simulink model "SwingUp_LQR"  (R2016a)
settings: Solver=VariableStepAuto  StartTime=0.0  StopTime=30  RelTol=1e-3
undefined symbols (not defined in the file): K1, K2, K3, K4
libraries: simulink x2, instrumentlib x2
settings Model: Creator=VILLOTA  LastModifiedBy=VILLOTA

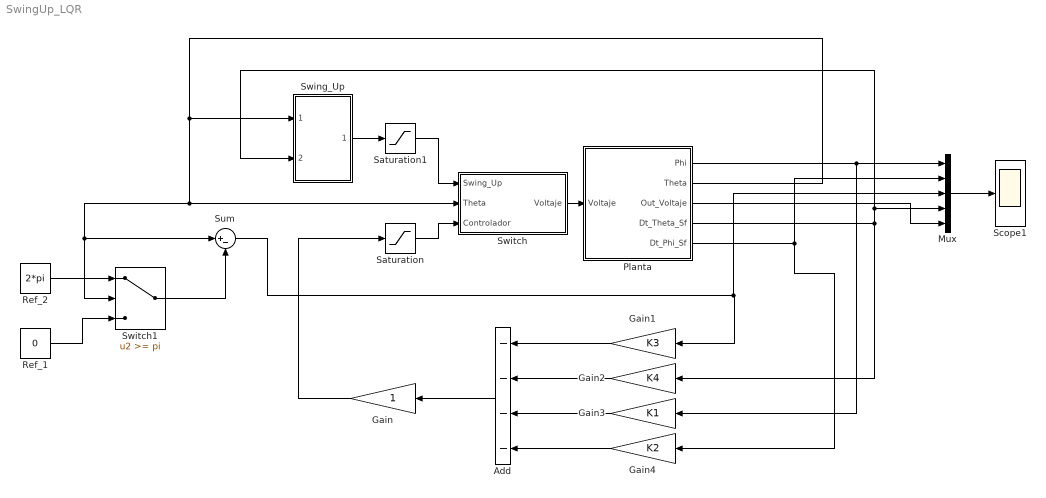
== system SwingUp_LQR ==
  Add : Sum  Inputs=----
  Gain : Gain
  Gain1 : Gain  Gain=K3
  Gain2 : Gain  Gain=K4
  Gain3 : Gain  Gain=K1
  Gain4 : Gain  Gain=K2
  Mux : Mux  Inputs=5
  Planta : Subsystem
  Ref_1 : Constant  Value=0
  Ref_2 : Constant  Value=2*pi
  Saturation : Saturate  UpperLimit=5  LowerLimit=-5
  Saturation1 : Saturate  UpperLimit=5  LowerLimit=-5
  Scope1 : Scope
  Sum : Sum  Inputs=|+-
  Swing_Up : Subsystem
  Switch : Subsystem
  Switch1 : Switch  Threshold=pi
  wires:
  Switch/1(Voltaje) -> Planta/1(Voltaje)
  Saturation/1 -> Switch/3(Controlador)
  Swing_Up/1(Voltaje) -> Saturation1/1
  Ref_2/1 -> Switch1/1
  Switch1/1 -> Sum/2
  Ref_1/1 -> Switch1/3
  Planta/2(Theta) -> Swing_Up/1(Theta), Switch1/2, Sum/1, Switch/2(Theta)
  Gain/1 -> Saturation/1
  Saturation1/1 -> Switch/1(Swing_Up)
  Add/1 -> Gain/1
  Sum/1 -> Mux/3, Gain1/1
  Planta/4(Dt_Theta_Sf) -> Gain2/1, Mux/4, Swing_Up/2(Theta')
  Planta/1(Phi) -> Mux/1, Gain3/1
  Gain2/1 -> Add/2
  Gain1/1 -> Add/1
  Gain3/1 -> Add/3
  Gain4/1 -> Add/4
  Planta/5(Dt_Phi_Sf) -> Mux/2, Gain4/1
  Planta/3(Out_Voltaje) -> Mux/5
  Mux/1 -> Scope1/1

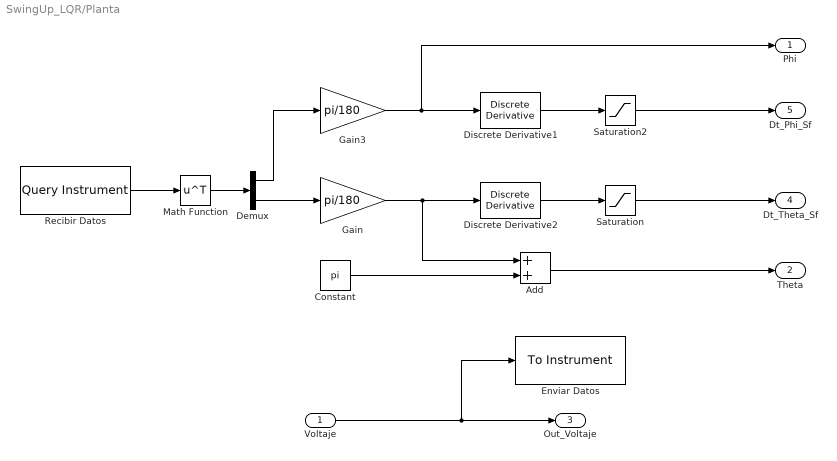
== system SwingUp_LQR/Planta ==
  Voltaje : Inport
  Add : Sum
  Constant : Constant  Value=pi
  Demux : Demux  Outputs=2
  Discrete Derivative1 : simulink/Discrete/Discrete Derivative  gainval=1.0  ICPrevScaledInput=0.0  OutMin=[]  OutMax=[]  OutDataType=fixdt(1, 16)  OutScaling=2^-10  DoSatur=off
  Discrete Derivative2 : simulink/Discrete/Discrete Derivative  gainval=1.0  ICPrevScaledInput=0.0  OutMin=[]  OutMax=[]  OutDataType=fixdt(1, 16)  OutScaling=2^-10  DoSatur=off
  Enviar Datos : instrumentlib/To Instrument  sampleTime=0.01  isWorkspaceObject=off  timeout=5  inputBufferSize=8192  protocol=Serial  serialPort=COM3  baudRate=115200  gpibVendor=Agilent Technologies  boardIndex=0  primaryAddress=1  secondaryAddress=0  visaVendor=Agilent  visaSerialPort=0  chassisIndex=0  logicalAddress=0  tcpRemoteHost='127.0.0.1'  tcpRemotePort=4500  udpRemoteHost='127.0.0.1'  udpRemotePort=9090  visaTCPBoardIndex=0  visaTCPRemoteHost='127.0.0.1'  usbBoardIndex=0  usbManufID=0  usbModelCode=0  usbSerialNumber=0  initAction=None  initCommand='a\n'  initFunction=get  command=''  sendFormat=ASCII  asciiFormatting='%f\n'  precision=8-bit integer  byteOrder=Little Endian
  Gain : Gain  Gain=pi/180
  Gain3 : Gain  Gain=pi/180
  Math Function : Math  Operator=transpose  SaturateOnIntegerOverflow=on
  Recibir Datos : instrumentlib/Query Instrument  sampleTime=0.01  isWorkspaceObject=off  timeout=5  inputBufferSize=512  protocol=Serial  serialPort=COM3  baudRate=115200  gpibVendor=Agilent Technologies  boardIndex=0  primaryAddress=1  secondaryAddress=0  visaVendor=Agilent  visaSerialPort=0  chassisIndex=0  logicalAddress=0  tcpRemoteHost='127.0.0.1'  tcpRemotePort=4500  udpRemoteHost='127.0.0.1'  udpRemotePort=9090  visaTCPBoardIndex=0  visaTCPRemoteHost='127.0.0.1'  usbBoardIndex=0  usbManufID=0  usbModelCode=0  usbSerialNumber=0  initAction=Send ASCII Commands  initCommand='%1'  initFunction=get  queryCommand=''  responseFormat=ASCII  asciiFormatting='%f,%f\r'  precision=8-bit integer  byteOrder=Little Endian  valuesToRead=1  removeBytes=on  afterOutputAction=Repeat query for new data  enableFrames=on  frameSize=2
  Saturation : Saturate  UpperLimit=40  LowerLimit=-40
  Saturation2 : Saturate  UpperLimit=40  LowerLimit=-40
  Phi : Outport
  Theta : Outport  Port=2
  Out_Voltaje : Outport  Port=3
  Dt_Theta_Sf : Outport  Port=4
  Dt_Phi_Sf : Outport  Port=5
  wires:
  Constant/1 -> Add/2
  Add/1 -> Theta/1
  Saturation/1 -> Dt_Theta_Sf/1
  Discrete Derivative2/1 -> Saturation/1
  Demux/2 -> Gain/1
  Math Function/1 -> Demux/1
  Recibir Datos/1 -> Math Function/1
  Gain/1 -> Discrete Derivative2/1, Add/1
  Voltaje/1 -> Enviar Datos/1, Out_Voltaje/1
  Saturation2/1 -> Dt_Phi_Sf/1
  Discrete Derivative1/1 -> Saturation2/1
  Demux/1 -> Gain3/1
  Gain3/1 -> Phi/1, Discrete Derivative1/1

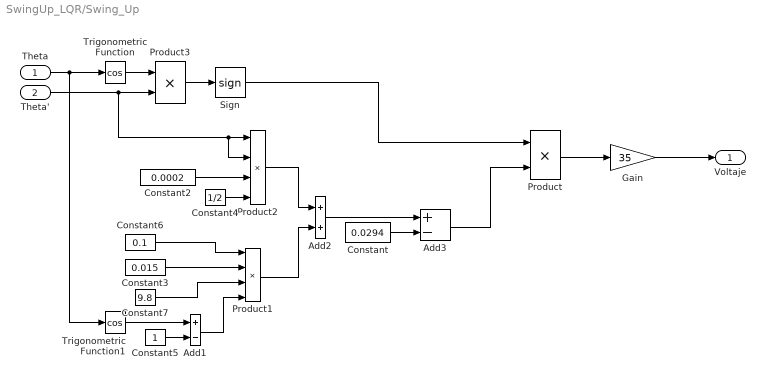
== system SwingUp_LQR/Swing_Up ==
  Theta : Inport
  Theta' : Inport  Port=2
  Add1 : Sum  Inputs=+-
  Add2 : Sum
  Add3 : Sum  Inputs=+-
  Constant : Constant  Value=0.0294
  Constant2 : Constant  Value=0.0002
  Constant3 : Constant  Value=0.015
  Constant4 : Constant  Value=1/2
  Constant5 : Constant
  Constant6 : Constant  Value=0.1
  Constant7 : Constant  Value=9.8
  Gain : Gain  Gain=35
  Product : Product
  Product1 : Product  Inputs=4
  Product2 : Product  Inputs=4
  Product3 : Product
  Sign : Signum
  Trigonometric Function : Trigonometry  Operator=cos
  Trigonometric Function1 : Trigonometry  Operator=cos
  Voltaje : Outport
  wires:
  Theta/1 -> Trigonometric Function/1, Trigonometric Function1/1
  Trigonometric Function/1 -> Product3/1
  Product3/1 -> Sign/1
  Constant3/1 -> Product1/2
  Constant6/1 -> Product1/1
  Constant4/1 -> Product2/4
  Constant7/1 -> Product1/3
  Trigonometric Function1/1 -> Add1/1
  Constant5/1 -> Add1/2
  Product2/1 -> Add2/1
  Product1/1 -> Add2/2
  Add2/1 -> Add3/1
  Sign/1 -> Product/1
  Product/1 -> Gain/1
  Constant/1 -> Add3/2
  Theta'/1 -> Product2/2, Product2/1, Product3/2
  Add1/1 -> Product1/4
  Add3/1 -> Product/2
  Gain/1 -> Voltaje/1
  Constant2/1 -> Product2/3

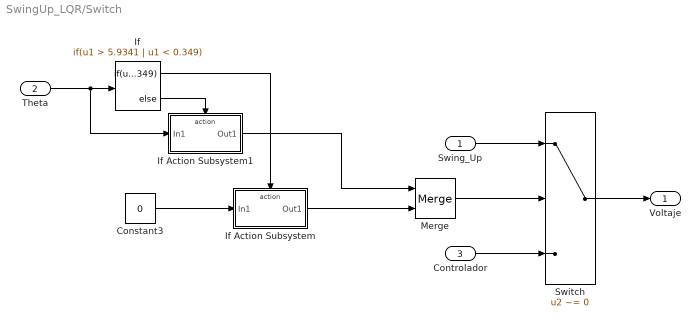
== system SwingUp_LQR/Switch ==
  Swing_Up : Inport
  Theta : Inport  Port=2
  Controlador : Inport  Port=3
  Constant3 : Constant  Value=0
  If : If  IfExpression=u1 > 5.9341 | u1 < 0.349
  If Action Subsystem : Subsystem  TreatAsAtomicUnit=on
  If Action Subsystem1 : Subsystem  TreatAsAtomicUnit=on
  Merge : Merge
  Switch : Switch  Criteria=u2 ~= 0  Threshold=(15*pi)/180
  Voltaje : Outport
  wires:
  Controlador/1 -> Switch/3
  Theta/1 -> If/1, If Action Subsystem1/1(In1)
  If Action Subsystem/1(Out1) -> Merge/2
  Swing_Up/1 -> Switch/1
  Constant3/1 -> If Action Subsystem/1(In1)
  Switch/1 -> Voltaje/1
  Merge/1 -> Switch/2
  If/2 -> If Action Subsystem1/Action
  If/1 -> If Action Subsystem/Action
  If Action Subsystem1/1(Out1) -> Merge/1

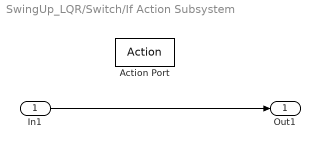
== system SwingUp_LQR/Switch/If Action Subsystem ==
  In1 : Inport
  Action Port : ActionPort  ActionType=then
  Out1 : Outport
  wires:
  In1/1 -> Out1/1

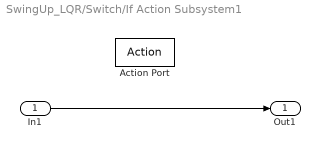
== system SwingUp_LQR/Switch/If Action Subsystem1 ==
  In1 : Inport
  Action Port : ActionPort  ActionType=else
  Out1 : Outport
  wires:
  In1/1 -> Out1/1
